simulink library "MusicLimiterLib"  (R2022b)
settings: Solver=VariableStepAuto  StartTime=0.0  StopTime=10.0  RelTol=1e-3
undefined symbols (not defined in the file or in its folder): Row
libraries: TuneVar x13, TOP x6, HandyTextFile x2, AudioStats x1, FeaturePath x1
settings Model: Creator=jb1046154  LastModifiedBy=sa1045272
settings SolverCC: AlgebraicLoopSolver=TrustRegion
settings DataIOCC: ReturnWorkspaceOutputs=off
settings DebuggingCC: UnconnectedInputMsg=warning  UnconnectedOutputMsg=warning  UnconnectedLineMsg=warning  SFMachineParentedDataDiag=warning  ArithmeticOperatorsInVariantConditions=warning
settings ModelReferenceCC: EnableRefExpFcnMdlSchedulingChecks=on
settings SFSimCC: CustomCodeUndefinedFunction=UseInterfaceOnly

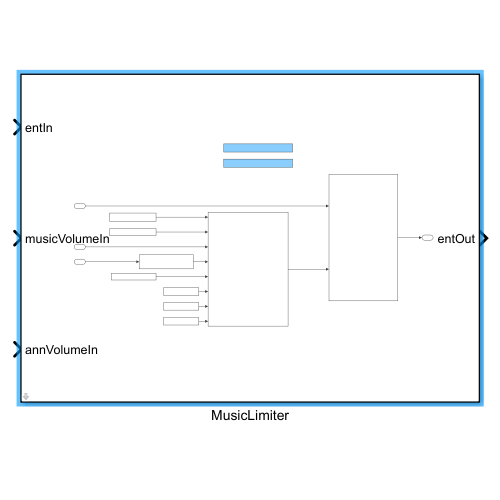
[thumbnail: Simulink's stored preview of the top-level diagram]
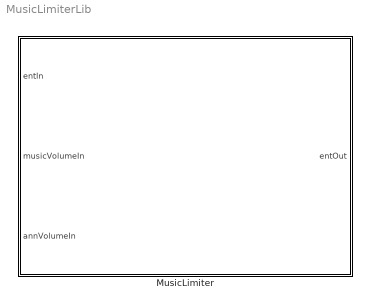
== system MusicLimiterLib ==
  MusicLimiter : Subsystem  mask(MusicLimiter){Config=[]}
      mask prompts: Config "MusicLimiterConfig"
      mask help:
      | This mask allows the setting of parameters for the MusicLimiter model.
      | Model parameters are set by a class instance in the base workspace.
      |
      | See 'Help' for details.
      mask init:
      | blkh=gcbh;
      | Config=BTConfig.Assert(blkh,Config);
      | 
      | Config.Validate();
      | Config.DoMaskInit(blkh);
      mask Help:
      | Defining model parameters:
      | The model parameters are set by the conents of an instance of MusicLimiterClass.m.
      | 
      | To set model parameters:
      | 1-Create an instance of MusicLimiterClass.m in the base workspace.
      | 2-In the model mask, set the 'Class instance' parameter to the name of the class instance in the base workspace.

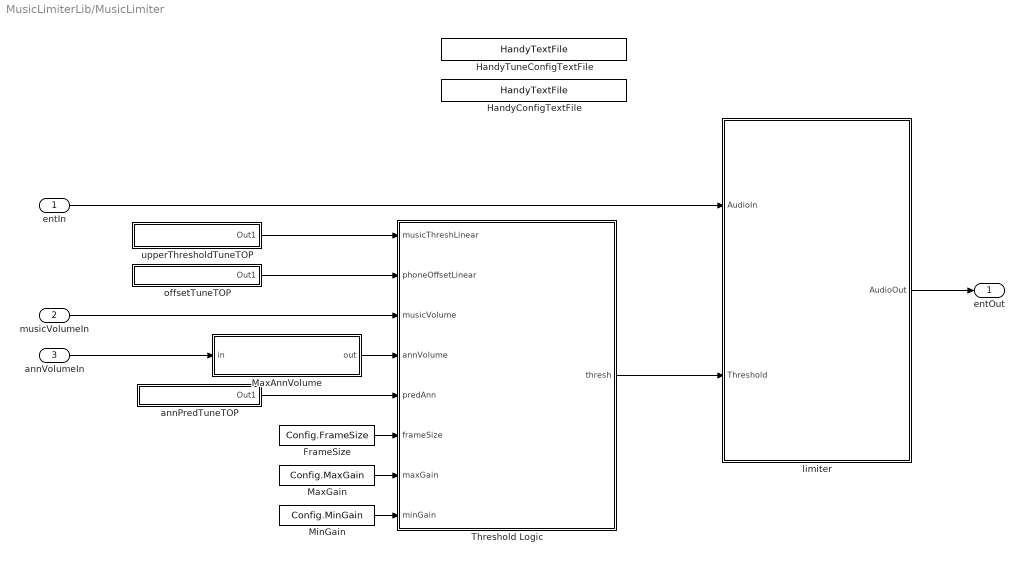
== system MusicLimiterLib/MusicLimiter ==
  entIn : Inport
  musicVolumeIn : Inport  Port=2
  annVolumeIn : Inport  Port=3
  FrameSize : Constant  Value=Config.FrameSize
  HandyConfigTextFile : HandyTextFile/HandyTextFile  TemplateSource=Config  FileSuffix=File  OpenDialogOnLoad=off  UseThisBlockName=off  AddGrandParentNamePrefix=off  TheDefaultText=% $(FILENAME) $(PREFIX) $(SUFFIX)  ShowInLibBrowser=on
      settings: SourceProductName=Bose Talaria
  HandyTuneConfigTextFile : HandyTextFile/HandyTextFile  TemplateSource=TuneConfig  FileSuffix=File  OpenDialogOnLoad=off  UseThisBlockName=off  AddGrandParentNamePrefix=off  TheDefaultText=% $(FILENAME) $(PREFIX) $(SUFFIX)  ShowInLibBrowser=on
      settings: SourceProductName=Bose Talaria
  MaxAnnVolume : MATLAB Function
  MaxGain : Constant  Value=Config.MaxGain
  MinGain : Constant  Value=Config.MinGain
  Threshold Logic : MATLAB Function
  annPredTuneTOP : Subsystem
  limiter : Subsystem
      mask DialogControl Container3 Prompt: Parameter Set
      mask Display:
      | [path,w,h] = IconLimiterMask();
      | 
      | % work in pixels since the icon does not scale
      | pos = get(gcbh,'position');
      | bw = pos(3) - pos(1);
      | bh = pos(4) - pos(2);
      | 
      | % Draw centered icon
      | xAdj = bw/2 - w/2;
      | yAdj = bh/2 - h/2 + 4;
      | for i=1:length(path)
      |     if (path(i).rgb(1) >= 0)
      |         patch(path(i).x+xAdj, path(i).y+yAdj, path(i).rgb);
      |     end
      |     if (path(i).stroke(1) >= 0)
      |         plot(path(i).x+xAdj, path(i).y+yAdj);
      |     end
      | end
      | 
      | % Anchor the corners of the coordinate system
      | patch(0,0,[1 1 1]);
      | patch(bw,bh,[1 1 1]);
      | 
      | % Display some text
      | text(bw/2, 4,'Limiter', ...
      |     'horizontalAlignment','center', ...
      |     'VerticalAlignment','bottom');
  offsetTuneTOP : Subsystem
  upperThresholdTuneTOP : Subsystem
  entOut : Outport  VectorParamsAs1DForOutWhenUnconnected=off
  wires:
  entIn/1 -> limiter/1(AudioIn)
  Threshold Logic/1(thresh) -> limiter/2(Threshold)
  limiter/1(AudioOut) -> entOut/1
  FrameSize/1 -> Threshold Logic/6(frameSize)
  musicVolumeIn/1 -> Threshold Logic/3(musicVolume)
  annVolumeIn/1 -> MaxAnnVolume/1(in)
  MaxAnnVolume/1(out) -> Threshold Logic/4(annVolume)
  upperThresholdTuneTOP/1(Out1) -> Threshold Logic/1(musicThreshLinear)
  offsetTuneTOP/1(Out1) -> Threshold Logic/2(phoneOffsetLinear)
  annPredTuneTOP/1(Out1) -> Threshold Logic/5(predAnn)
  MaxGain/1 -> Threshold Logic/7(maxGain)
  MinGain/1 -> Threshold Logic/8(minGain)

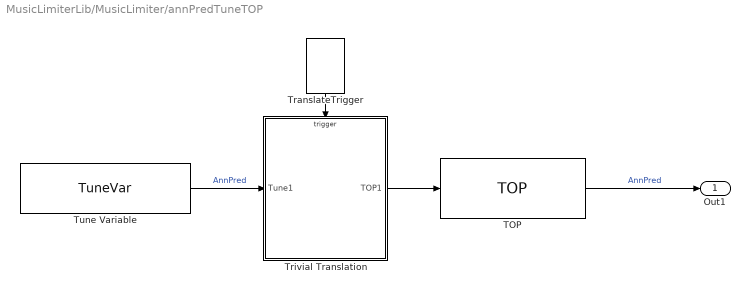
== system MusicLimiterLib/MusicLimiter/annPredTuneTOP ==
  TOP : TOP/TOP  TriggerInit=[440 20 585 80]  TopName=AnnPred  DataType=single  BankNumber=0  PreOverlay=false  PostOverlay=false  Role=Automatic
      settings: SourceProductName=Bose Talaria
  TranslateTrigger : TuneVar/TranslateTrigger  TriggerInit=[306 -100 344 -45]
      settings: SourceProductName=Bose Talaria
  Trivial Translation : MATLAB Function  TreatAsAtomicUnit=on
  Tune Variable : TuneVar/TuneVar  TuneName=AnnPred  SpecifyMaxSize=off  VariableDim=1 (Row)  MaxSize=[1 1]  TunabilityNumber=1  MinValue=[]  MaxValue=[]  TriggerInit=[20 25 190 75]  MaskValue=Config.TuneDefaults.AnnPred
      settings: SourceProductName=Bose Talaria
  Out1 : Outport  VectorParamsAs1DForOutWhenUnconnected=off
  wires:
  TOP/1 -> Out1/1  "AnnPred"
  Tune Variable/1 -> Trivial Translation/1(Tune1)  "AnnPred"
  Trivial Translation/1(TOP1) -> TOP/1
  TranslateTrigger/1 -> Trivial Translation/Trigger

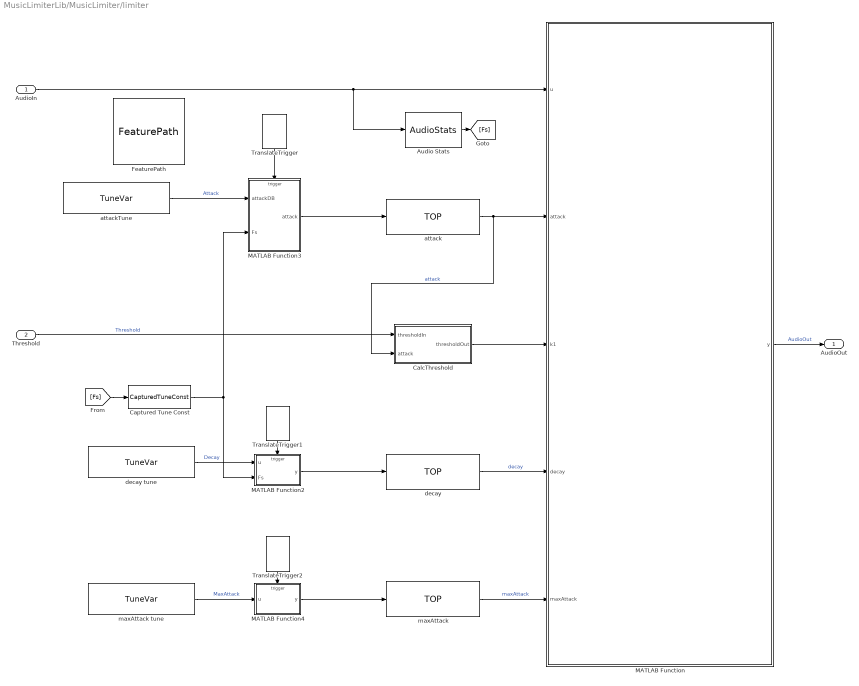
== system MusicLimiterLib/MusicLimiter/limiter ==
  AudioIn : Inport
  Threshold : Inport  Port=2
  Audio Stats : AudioStats/AudioStats  DoSampleRate=on  TypeSampleRate=double  DoCallRate=off  TypeCallRate=Inherit: auto  DoFrameSize=off  TypeFrameSize=Inherit: auto  DoChannelCount=off  TypeChannelCount=Inherit: auto  DoTaskRateFactor=off  TypeTaskRateFactor=Inherit: auto  MacroNameRoot=AUDIO  MacroNameRootEval='AUDIO'  IsMacroNameEval=off  MacroSampleRate=off  MacroCallRate=off  MacroFrameSize=off  MacroChannelCount=off  MacroTaskRateFactor=off  MacroTaskId=off  ValidateSampleRate=off  ValueSampleRate=[]  ValidateCallRate=off  ValueCallRate=[]  ValidateFrameSize=off  ValueFrameSize=[]  ValidateChannelCount=off  ValueChannelCount=[]  ValidateTaskRateFactor=off  ValueTaskRateFactor=[]
      settings: SourceProductName=Bose Talaria
  CalcThreshold : MATLAB Function  TreatAsAtomicUnit=on
  Captured Tune Const : TuneVar/CapturedTuneConst  TriggerInit=[45 452 145 488]  Role=Automatic
      settings: SourceProductName=Bose Talaria
  FeaturePath : FeaturePath/FeaturePath  FeatureName=Limiter  IsGroup=off  GroupNumber=-1  IsModule=off  TriggerInit=[20 -11 135 96]
      settings: SourceProductName=Bose Talaria
  MATLAB Function : MATLAB Function  TreatAsAtomicUnit=on
  MATLAB Function2 : MATLAB Function  TreatAsAtomicUnit=on
  MATLAB Function3 : MATLAB Function  TreatAsAtomicUnit=on
  MATLAB Function4 : MATLAB Function  TreatAsAtomicUnit=on
  TranslateTrigger : TuneVar/TranslateTrigger  TriggerInit=[261 15 299 70]
      settings: SourceProductName=Bose Talaria
  TranslateTrigger1 : TuneVar/TranslateTrigger  TriggerInit=[266 485 304 540]
      settings: SourceProductName=Bose Talaria
  TranslateTrigger2 : TuneVar/TranslateTrigger  TriggerInit=[266 695 304 750]
      settings: SourceProductName=Bose Talaria
  attack : TOP/TOP  TriggerInit=[460 152 610 208]  TopName=attack  DataType=single  BankNumber=0  PreOverlay=false  PostOverlay=false  Role=Automatic
      settings: SourceProductName=Bose Talaria
  attackTune : TuneVar/TuneVar  TuneName=Attack  SpecifyMaxSize=off  VariableDim=1 (Row)  MaxSize=[1 1]  TunabilityNumber=1  MinValue=[]  MaxValue=[]  TriggerInit=[-60 125 110 175]  MaskValue=Config.TuneDefaults.LimiterAttack
      settings: SourceProductName=Bose Talaria
  decay : TOP/TOP  TriggerInit=[460 562 610 618]  TopName=decay  DataType=single  BankNumber=0  PreOverlay=false  PostOverlay=false  Role=Automatic
      settings: SourceProductName=Bose Talaria
  decay tune : TuneVar/TuneVar  TuneName=Decay  SpecifyMaxSize=off  VariableDim=1 (Row)  MaxSize=[1 1]  TunabilityNumber=1  MinValue=[]  MaxValue=[]  TriggerInit=[-20 550 150 600]  MaskValue=Config.TuneDefaults.LimiterDecay
      settings: SourceProductName=Bose Talaria
  maxAttack : TOP/TOP  TriggerInit=[460 767 610 823]  TopName=maxAttack  DataType=single  BankNumber=0  PreOverlay=false  PostOverlay=false  Role=Automatic
      settings: SourceProductName=Bose Talaria
  maxAttack tune : TuneVar/TuneVar  TuneName=MaxAttack  SpecifyMaxSize=off  VariableDim=1 (Row)  MaxSize=[1 1]  TunabilityNumber=1  MinValue=[]  MaxValue=[]  TriggerInit=[-20 770 150 820]  MaskValue=Config.TuneDefaults.LimiterMaxAttack
      settings: SourceProductName=Bose Talaria
  AudioOut : Outport  VectorParamsAs1DForOutWhenUnconnected=off
  wires:
  Captured Tune Const/1 -> MATLAB Function2/2(Fs), MATLAB Function3/2(Fs)
  MATLAB Function3/1(attack) -> attack/1
  maxAttack/1 -> MATLAB Function/5(maxAttack)  "maxAttack"
  MATLAB Function4/1(y) -> maxAttack/1
  TranslateTrigger2/1 -> MATLAB Function4/Trigger
  maxAttack tune/1 -> MATLAB Function4/1(u)  "MaxAttack"
  TranslateTrigger/1 -> MATLAB Function3/Trigger
  [Fs] -> Captured Tune Const/1
  Audio Stats/1 -> [Fs]
  decay/1 -> MATLAB Function/4(decay)  "decay"
  MATLAB Function2/1(y) -> decay/1
  attack/1 -> CalcThreshold/2(attack), MATLAB Function/2(attack)  "attack"
  TranslateTrigger1/1 -> MATLAB Function2/Trigger
  decay tune/1 -> MATLAB Function2/1(u)  "Decay"
  attackTune/1 -> MATLAB Function3/1(attackDB)  "Attack"
  MATLAB Function/1(y) -> AudioOut/1  "AudioOut"
  AudioIn/1 -> Audio Stats/1, MATLAB Function/1(u)
  CalcThreshold/1(thresholdOut) -> MATLAB Function/3(k1)
  Threshold/1 -> CalcThreshold/1(thresholdIn)  "Threshold"

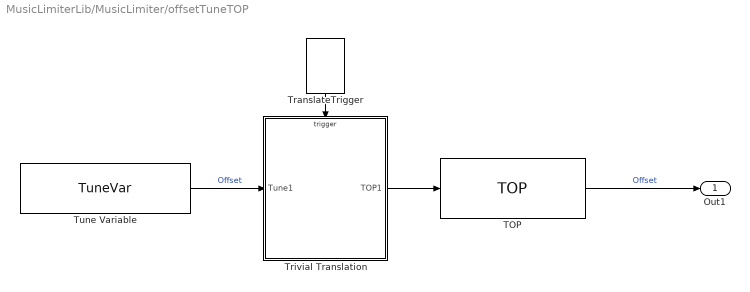
== system MusicLimiterLib/MusicLimiter/offsetTuneTOP ==
  TOP : TOP/TOP  TriggerInit=[440 20 585 80]  TopName=Offset  DataType=single  BankNumber=0  PreOverlay=false  PostOverlay=false  Role=Automatic
      settings: SourceProductName=Bose Talaria
  TranslateTrigger : TuneVar/TranslateTrigger  TriggerInit=[306 -100 344 -45]
      settings: SourceProductName=Bose Talaria
  Trivial Translation : MATLAB Function  TreatAsAtomicUnit=on
  Tune Variable : TuneVar/TuneVar  TuneName=Offset  SpecifyMaxSize=off  VariableDim=1 (Row)  MaxSize=[1 1]  TunabilityNumber=1  MinValue=[]  MaxValue=[]  TriggerInit=[20 25 190 75]  MaskValue=Config.TuneDefaults.Offset
      settings: SourceProductName=Bose Talaria
  Out1 : Outport  VectorParamsAs1DForOutWhenUnconnected=off
  wires:
  TOP/1 -> Out1/1  "Offset"
  Tune Variable/1 -> Trivial Translation/1(Tune1)  "Offset"
  Trivial Translation/1(TOP1) -> TOP/1
  TranslateTrigger/1 -> Trivial Translation/Trigger

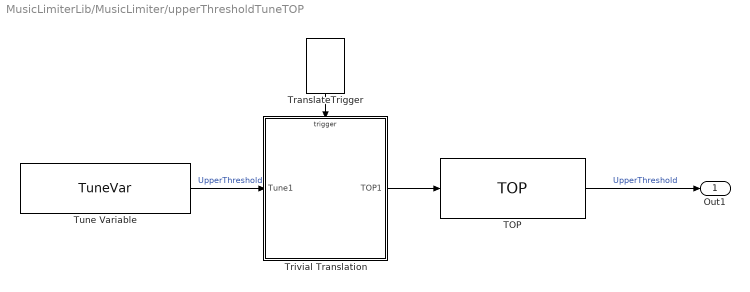
== system MusicLimiterLib/MusicLimiter/upperThresholdTuneTOP ==
  TOP : TOP/TOP  TriggerInit=[440 20 585 80]  TopName=UpperThreshold  DataType=single  BankNumber=0  PreOverlay=false  PostOverlay=false  Role=Automatic
      settings: SourceProductName=Bose Talaria
  TranslateTrigger : TuneVar/TranslateTrigger  TriggerInit=[306 -100 344 -45]
      settings: SourceProductName=Bose Talaria
  Trivial Translation : MATLAB Function  TreatAsAtomicUnit=on
  Tune Variable : TuneVar/TuneVar  TuneName=UpperThreshold  SpecifyMaxSize=off  VariableDim=1 (Row)  MaxSize=[1 1]  TunabilityNumber=1  MinValue=[]  MaxValue=[]  TriggerInit=[20 25 190 75]  MaskValue=Config.TuneDefaults.UpperThreshold
      settings: SourceProductName=Bose Talaria
  Out1 : Outport  VectorParamsAs1DForOutWhenUnconnected=off
  wires:
  TOP/1 -> Out1/1  "UpperThreshold"
  Tune Variable/1 -> Trivial Translation/1(Tune1)  "UpperThreshold"
  Trivial Translation/1(TOP1) -> TOP/1
  TranslateTrigger/1 -> Trivial Translation/Trigger

== matlab function MusicLimiterLib/MusicLimiter/MaxAnnVolume ==
  data: in input; out output
function out = max_ann_volume(in)

out = single(ones(1,32));
for idx = 1:size(in, 2)
    out(idx) = max(in(:, idx));
end

== matlab function MusicLimiterLib/MusicLimiter/offsetTuneTOP/Trivial Translation ==
  data: TOP1 output; Tune1 input
  events: trigger input FUNCTION_CALL_EVENT
function TOP1  = fcn(Tune1)
%#codegen

% ----- To access TuneVar maximum size, current size, and current value:
%   Note: TuneVar signals arrive with exposed variable size information.
%         The expressions below illustrate for the "Tune1" input argument.
%
%   size(Tune1.Value) : the maximum possible size of the Tune1 variable
%
%   Tune.Size   : the current size of *valid* data in Tune1.Value
%
%   Tune1.Size(1) : Number of rows present in Tune1 - this does not vary.
%
%   Tune1.Size(2) : Number of columns currently valid in Tune1 - this is
%       the variable part of size that can change (if allowed by TuneVar).
%
%   Tune1.Value : the current value of the tune variable... but end-padded 
%       to the maximum available size with undefined/invalid data.
%
%   numel(Tune1.Value) : another way of looking at the maximum number of
%       elements that could arrive in Tune1.Value
%
% ----- To register an error, use the following method (works like printf):
%   TranslateError( <format string>, <arguments ... )
%   ... this error will cause the build process to abort.

% A trivial pass-through translation looks like this:
%TOP1 = Tune1.Value;
TOP1 = 10 ^ ((Tune1.Value) / 20);

== matlab function MusicLimiterLib/MusicLimiter/limiter/MATLAB Function ==
  data: u input; y output; attack input; k1 input; decay input; maxAttack input
function y = limiter(u, attack, k1, decay, maxAttack)

% Grab data from input
y = coder.nullcopy(u);
[frameSize, channelCount] = size(u);

maxGain = single(1);

persistent state;
if isempty(state)
    state = single(1 * ones(1,channelCount));
end

% Process the audio
for i = 1:channelCount
    k0 = 1 + attack(i);
    g1 = state(i);

    for s = 1:frameSize
        % Compute the gain for this sample. Implementation copied from BDSP
        p1 = k1(i) * g1;
        p2 = u(s, i);
        p2 = abs(p2);
        g1 = g1 * decay(i);
        p2 = p2 * p1;
        p2 = max(p2, attack(i));
        p2 = k0 - p2;
        p2 = max(p2, maxAttack(i));
        g1 = g1 * p2;
        g1 = min(g1, maxGain);

        % Apply the gain
        y(s, i) = u(s, i) * g1;
    end

    state(i) = g1;
end

== matlab function MusicLimiterLib/MusicLimiter/annPredTuneTOP/Trivial Translation ==
  data: TOP1 output; Tune1 input
  events: trigger input FUNCTION_CALL_EVENT
function TOP1  = fcn(Tune1)
%#codegen

% ----- To access TuneVar maximum size, current size, and current value:
%   Note: TuneVar signals arrive with exposed variable size information.
%         The expressions below illustrate for the "Tune1" input argument.
%
%   size(Tune1.Value) : the maximum possible size of the Tune1 variable
%
%   Tune.Size   : the current size of *valid* data in Tune1.Value
%
%   Tune1.Size(1) : Number of rows present in Tune1 - this does not vary.
%
%   Tune1.Size(2) : Number of columns currently valid in Tune1 - this is
%       the variable part of size that can change (if allowed by TuneVar).
%
%   Tune1.Value : the current value of the tune variable... but end-padded 
%       to the maximum available size with undefined/invalid data.
%
%   numel(Tune1.Value) : another way of looking at the maximum number of
%       elements that could arrive in Tune1.Value
%
% ----- To register an error, use the following method (works like printf):
%   TranslateError( <format string>, <arguments ... )
%   ... this error will cause the build process to abort.

% A trivial pass-through translation looks like this:
%TOP1 = Tune1.Value;
TOP1 = 10 ^ ((Tune1.Value) / 20);

== matlab function MusicLimiterLib/MusicLimiter/limiter/MATLAB Function2 ==
  data: u input; y output; Fs input
  events: trigger input FUNCTION_CALL_EVENT
function y = fcn(u, Fs)

y = single(undb20(abs(u.Value) / Fs));

== matlab function MusicLimiterLib/MusicLimiter/limiter/MATLAB Function3 ==
  data: attackDB input; Fs input; attack output
  events: trigger input FUNCTION_CALL_EVENT
%function [attack, k1]= fcn(attackDB, threshold, Fs)
function attack = fcn(attackDB, Fs)
attack = single(1 - undb20(-abs(attackDB.Value) / Fs));
%k1 = attack ./ single(threshold.Value);

== matlab function MusicLimiterLib/MusicLimiter/limiter/MATLAB Function4 ==
  data: u input; y output
  events: trigger input FUNCTION_CALL_EVENT
function y = fcn(u)

y = single(undb20(-abs(u.Value)));

== matlab function MusicLimiterLib/MusicLimiter/limiter/CalcThreshold ==
  data: thresholdIn input; thresholdOut output; attack input
function thresholdOut = calcThreshold(thresholdIn, attack)

thresholdOut = attack ./ single(thresholdIn);

== matlab function MusicLimiterLib/MusicLimiter/upperThresholdTuneTOP/Trivial Translation ==
  data: TOP1 output; Tune1 input
  events: trigger input FUNCTION_CALL_EVENT
function TOP1  = fcn(Tune1)
%#codegen

% ----- To access TuneVar maximum size, current size, and current value:
%   Note: TuneVar signals arrive with exposed variable size information.
%         The expressions below illustrate for the "Tune1" input argument.
%
%   size(Tune1.Value) : the maximum possible size of the Tune1 variable
%
%   Tune.Size   : the current size of *valid* data in Tune1.Value
%
%   Tune1.Size(1) : Number of rows present in Tune1 - this does not vary.
%
%   Tune1.Size(2) : Number of columns currently valid in Tune1 - this is
%       the variable part of size that can change (if allowed by TuneVar).
%
%   Tune1.Value : the current value of the tune variable... but end-padded 
%       to the maximum available size with undefined/invalid data.
%
%   numel(Tune1.Value) : another way of looking at the maximum number of
%       elements that could arrive in Tune1.Value
%
% ----- To register an error, use the following method (works like printf):
%   TranslateError( <format string>, <arguments ... )
%   ... this error will cause the build process to abort.

% A trivial pass-through translation looks like this:
%TOP1 = Tune1.Value;
TOP1 = 10 ^ ((Tune1.Value) / 20);

== matlab function MusicLimiterLib/MusicLimiter/Threshold Logic ==
  data: musicThreshLinear input; phoneOffsetLinear input; thresh output; musicVolume input; annVolume input; predAnn input; frameSize input; maxGain input; minGain input
function thresh  = threshCalc(musicThreshLinear, phoneOffsetLinear, musicVolume, annVolume, predAnn, frameSize, maxGain, minGain)
% Keep the music limited to the minimum of the specifed music threshold or
% the current level of the phone minus a tuned offset

thresh = single(annVolume);

% Limit announcement and entertainment volumes to 1 or less
annVolumeLimited = min(1.0, annVolume);
musicVolumeLimited = min(1.0, musicVolume);

% Calculate target threshold
annTargetLevel = predAnn * annVolumeLimited / (phoneOffsetLinear + eps);
targetLevel = min(musicThreshLinear, annTargetLevel);
musicVolumeSamp = musicVolumeLimited(floor((0:(numel(targetLevel)-1)) / frameSize) + 1);
thresh = targetLevel ./ (musicVolumeSamp + eps);

% Check limits
thresh = thresh / musicThreshLinear;
thresh = min(maxGain, thresh);
thresh = max(minGain, thresh);
